simulink model "algebraic_loop_test"  (R2019b)
settings: Solver=ode4  StartTime=0.0  StopTime=10.0  FixedStep=0.001  RelTol=1e-3
settings Model: Creator=PD Banneheka  LastModifiedBy=PD Banneheka

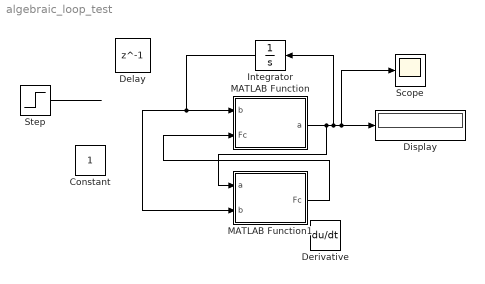
== system algebraic_loop_test ==
  Constant : Constant
  Delay : Delay  DelayLength=1
  Derivative : Derivative
  Display : Display
  Integrator : Integrator
  MATLAB Function : MATLAB Function  TreatAsAtomicUnit=on
  MATLAB Function1 : MATLAB Function  TreatAsAtomicUnit=on
  Scope : Scope
  Step : Step  Before=5  After=10  SampleTime=0
  wires:
  Step/1 -> ?
  MATLAB Function/1(a) -> MATLAB Function1/1(a), Integrator/1, Scope/1, Display/1
  Integrator/1 -> MATLAB Function/1(b), MATLAB Function1/2(b)
  MATLAB Function1/1(Fc) -> MATLAB Function/2(Fc)

== matlab function algebraic_loop_test/MATLAB Function1 ==
  data: a input; b input; Fc output
function Fc  = fcn(a,b)

Fc = a*b;

== matlab function algebraic_loop_test/MATLAB Function ==
  data: b input; Fc input; a output
function a  = fcn(b,Fc)

F = 5*b;

a = (F + Fc)/5;
